simulink model "ayaz_th"  (R2018b)
settings: Solver=ode15s  StartTime=0.0  StopTime=duration_s  MaxStep=5  RelTol=1e-3  AbsTol=1e-3
undefined symbols (not defined in the file or in its folder): unstretched_l, X0
libraries: ayazPlant_cl x1, ayazController_cl x1, ayazWinches_cl x1
settings Model: Creator=mcobb  LastModifiedBy=mcobb

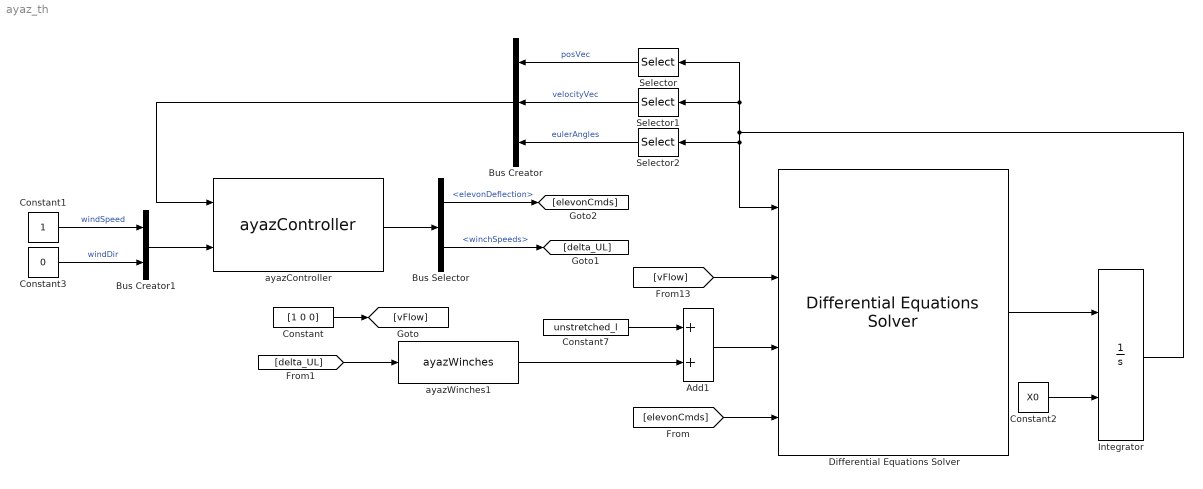
== system ayaz_th ==
  Add1 : Sum
  Bus Creator : BusCreator  Inputs=3  OutDataTypeStr=Bus: plantBus
  Bus Creator1 : BusCreator  Inputs=2  OutDataTypeStr=Bus: envBus
  Bus Selector : BusSelector  OutputSignals=elevonDeflection,winchSpeeds
  Constant : Constant  Value=[1 0 0]
  Constant1 : Constant
  Constant2 : Constant  Value=X0
  Constant3 : Constant  Value=0
  Constant7 : Constant  Value=unstretched_l
  Differential Equations Solver : ayazPlant_cl/ayazPlant/Differential Equations Solver  SystemSampleTime=-1
  Integrator : Integrator  InitialConditionSource=external  InitialCondition=X0
  Selector : Selector  InputPortWidth=50  IndexOptions=Index vector (dialog)  Indices=[1 2 3]  OutputSizes=1
  Selector1 : Selector  InputPortWidth=50  IndexOptions=Index vector (dialog)  Indices=[4 5 6]  OutputSizes=1
  Selector2 : Selector  InputPortWidth=50  IndexOptions=Index vector (dialog)  Indices=[7 8 9]  OutputSizes=1
  ayazController : ayazController_cl/ayazController  SystemSampleTime=-1  VariantControl=VSS_controller_ayazController
  ayazWinches1 : ayazWinches_cl/ayazWinches  SystemSampleTime=-1
  wires:
  [vFlow] -> Differential Equations Solver/2
  Integrator/1 -> Selector1/1, Selector/1, Selector2/1, Differential Equations Solver/1
  Constant2/1 -> Integrator/2
  [elevonCmds] -> Differential Equations Solver/4
  Constant7/1 -> Add1/1
  ayazWinches1/1 -> Add1/2
  Differential Equations Solver/1 -> Integrator/1
  Add1/1 -> Differential Equations Solver/3
  Constant/1 -> [vFlow]
  ayazController/1 -> Bus Selector/1
  Bus Selector/2 -> [delta_UL]  "<winchSpeeds>"
  Bus Selector/1 -> [elevonCmds]  "<elevonDeflection>"
  [delta_UL] -> ayazWinches1/1
  Bus Creator/1 -> ayazController/1
  Bus Creator1/1 -> ayazController/2
  Constant1/1 -> Bus Creator1/1  "windSpeed"
  Constant3/1 -> Bus Creator1/2  "windDir"
  Selector/1 -> Bus Creator/1  "posVec"
  Selector1/1 -> Bus Creator/2  "velocityVec"
  Selector2/1 -> Bus Creator/3  "eulerAngles"
